simulink model "friction_example_course"  (R2020b)
settings: Solver=VariableStepAuto  StartTime=0.0  StopTime=10.0  RelTol=1e-3
settings Model: Creator=TC16766  LastModifiedBy=TC16766

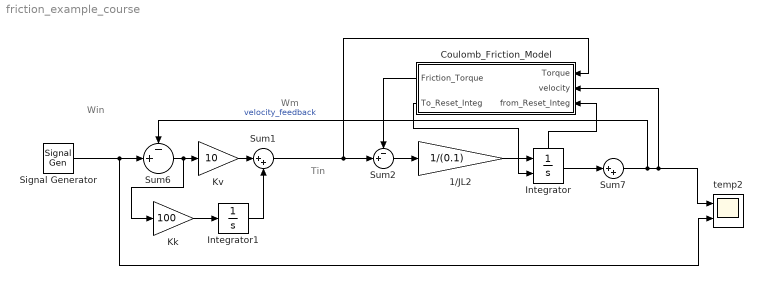
== system friction_example_course ==
  note: Tin
  note: Wm
  note: Win
  1/JL2 : Gain  Gain=1/(0.1)  SaturateOnIntegerOverflow=on  OutDataTypeStr=Inherit: Same as input  ParamDataTypeStr=Inherit: Same as input
  Coulomb_Friction_Model : Subsystem
  Integrator : Integrator  ExternalReset=rising  ShowStatePort=on
  Integrator1 : Integrator
  Kk : Gain  Gain=100  SaturateOnIntegerOverflow=on  OutDataTypeStr=Inherit: Same as input  ParamDataTypeStr=Inherit: Same as input
  Kv : Gain  Gain=10  SaturateOnIntegerOverflow=on  OutDataTypeStr=Inherit: Same as input  ParamDataTypeStr=Inherit: Same as input
  Signal Generator : SignalGenerator
  Sum1 : Sum  Inputs=|++  SaturateOnIntegerOverflow=on
  Sum2 : Sum  Inputs=-+|  SaturateOnIntegerOverflow=on
  Sum6 : Sum  Inputs=-+|  SaturateOnIntegerOverflow=on
  Sum7 : Sum  Inputs=|++  SaturateOnIntegerOverflow=on
  temp2 : Scope  NumInputPorts=2
  wires:
  Coulomb_Friction_Model/1(Friction_Torque) -> Sum2/1
  Integrator/1 -> Sum7/1
  Sum6/1 -> Kk/1, Kv/1
  1/JL2/1 -> Integrator/1
  Sum7/1 -> temp2/1, Coulomb_Friction_Model/2(velocity), Sum6/1  "velocity_feedback"
  Coulomb_Friction_Model/2(To_Reset_Integ) -> Integrator/2
  Sum2/1 -> 1/JL2/1
  Integrator/State -> Coulomb_Friction_Model/3(from_Reset_Integ)
  Signal Generator/1 -> Sum6/2, temp2/2
  Kv/1 -> Sum1/1
  Sum1/1 -> Sum2/2, Coulomb_Friction_Model/1(Torque)
  Integrator1/1 -> Sum1/2
  Kk/1 -> Integrator1/1

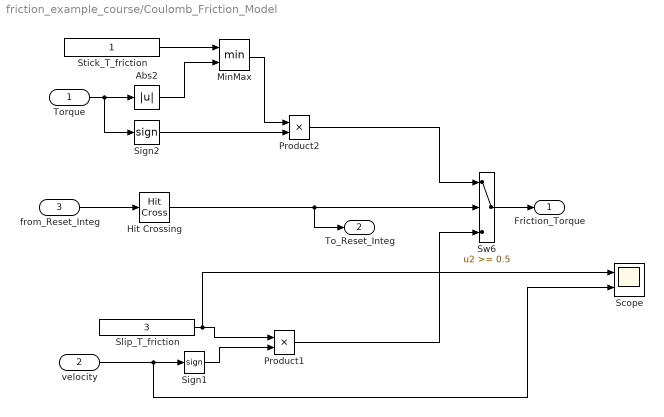
== system friction_example_course/Coulomb_Friction_Model ==
  Torque : Inport
  velocity : Inport  Port=2
  from_Reset_Integ : Inport  Port=3
  Abs2 : Abs
  Hit Crossing : HitCross  ZeroCross=off
  MinMax : MinMax  Inputs=2
  Product1 : Product  RndMeth=Zero
  Product2 : Product  RndMeth=Zero
  Scope : Scope  NumInputPorts=2
  Sign1 : Signum  ZeroCross=off
  Sign2 : Signum  ZeroCross=off
  Slip_T_friction : Constant  Value=3
  Stick_T_friction : Constant
  Sw6 : Switch  Threshold=0.5  SaturateOnIntegerOverflow=on  InputSameDT=on
  Friction_Torque : Outport
  To_Reset_Integ : Outport  Port=2
  wires:
  Torque/1 -> Abs2/1, Sign2/1
  Sw6/1 -> Friction_Torque/1
  velocity/1 -> Scope/2, Sign1/1
  Sign1/1 -> Product1/2
  Product1/1 -> Sw6/3
  Hit Crossing/1 -> To_Reset_Integ/1, Sw6/2
  from_Reset_Integ/1 -> Hit Crossing/1
  Sign2/1 -> Product2/2
  Stick_T_friction/1 -> MinMax/1
  Abs2/1 -> MinMax/2
  MinMax/1 -> Product2/1
  Product2/1 -> Sw6/1
  Slip_T_friction/1 -> Scope/1, Product1/1
